simulink model "PatientModelOL_DL"  (R2019b)
settings: Solver=VariableStepAuto  StartTime=0.0  StopTime=24*60  RelTol=1e-3
model workspace (MAT data in the model file):
  Cden = Simulink.Parameter
  Cden.Value = [0 0 0 0 0 0 0 0 0 1]
  Cden.DataType = 'auto'
  Cden.Dimensions = [1 10]
  Cnum = Simulink.Parameter
  Cnum.Value = [0 0 0 0 0 0 0 0 0 1]
  Cnum.DataType = 'auto'
  Cnum.Dimensions = [1 10]
  params = Simulink.Parameter
  params.Value = [1952.52414079 19.967779107 0.00715860498632 175.485035956 0.566549098404 0.00777036526415 0 14.6965723894 92.1976761985 158.929922349 168.789255183 0 0 0 0 0 0 0 0 0]
  params.DataType = 'auto'
  params.Dimensions = [1 20]
settings Model: Creator=vjoukov  LastModifiedBy=zaria
settings DataIOCC: ReturnWorkspaceOutputs=off
settings DebuggingCC: PregeneratedLibrarySubsystemCodeDiagnostic=none  ArithmeticOperatorsInVariantConditions=warning
settings SFSimCC: SimUseLocalCustomCode=off  CustomCodeUndefinedFunction=UseInterfaceOnly
settings RTWCC: RTWUseLocalCustomCode=off

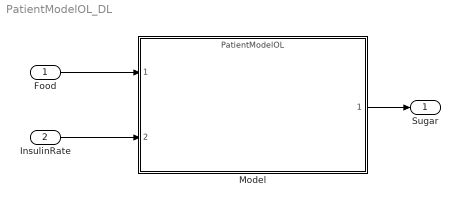
== system PatientModelOL_DL ==
  Food : Inport
  InsulinRate : Inport  Port=2
  Model : ModelReference  ModelNameDialog=PatientModelOL.slxp  ParameterArgumentNames=params  ParameterArgumentValues=params  UsingDefaultArgumentValue=0  ModelReferenceVersion=1.387  CopyOfModelProtected=on
  Sugar : Outport  VectorParamsAs1DForOutWhenUnconnected=off
  wires:
  Food/1 -> Model/1
  InsulinRate/1 -> Model/2
  Model/1 -> Sugar/1
